simulink library "simple_library"  (R2014a)
settings: Solver=ode45  StartTime=0.0  StopTime=10.0  RelTol=1e-3
settings Model: Creator=ladmin  LastModifiedBy=ladmin

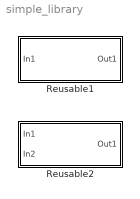
== system simple_library ==
  Reusable1 : Subsystem
  Reusable2 : Subsystem

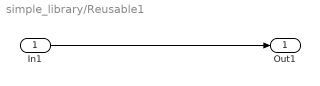
== system simple_library/Reusable1 ==
  In1 : Inport
  Out1 : Outport
  wires:
  In1/1 -> Out1/1

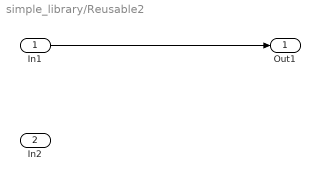
== system simple_library/Reusable2 ==
  In1 : Inport
  In2 : Inport  Port=2
  Out1 : Outport
  wires:
  In1/1 -> Out1/1
